simulink model "sldv_property2"  (R2015b)
settings: Solver=FixedStepDiscrete  SolverMode=SingleTasking  StartTime=0.0  StopTime=10.0  RelTol=1e-3
libraries: sldvlib x1
Description:
  | Model Coverage Test Generation
settings Model: Creator=The MathWorks Inc.  LastModifiedBy=amatsumo
settings DataIOCC: SaveFormat=Array  SignalLoggingSaveFormat=ModelDataLogs  SaveOutput=off  SignalLogging=off  SaveTime=off
settings OptimizationCC: BlockReduction=off  ConditionallyExecuteInputs=off  DefaultParameterBehavior=Inlined  ExpressionDepthLimit=2147483647  InitFltsAndDblsToZero=on  EfficientMapNaN2IntZero=off
settings DebuggingCC: AlgebraicLoopMsg=error  SaveWithParameterizedLinksMsg=none  UnderspecifiedInitializationDetection=Classic  MergeDetectMultiDrivingBlocksExec=none  SignalResolutionControl=TryResolveAllWithWarning  SolverPrmCheckMsg=warning  SingleTaskRateTransMsg=error  FcnCallInpInsideContextMsg=UseLocalSettings  StateNameClashWarn=warning
settings HardwareCC: ProdBitPerPointer=32  ProdLargestAtomicFloat=None  ProdIntDivRoundTo=Undefined  ProdEndianess=Unspecified  ProdWordSize=32  ProdHWDeviceType=ASIC/FPGA->ASIC/FPGA  ProdEqTarget=off
settings SFSimCC: SimParseCustomCode=off
settings GRTTargetCC: TargetFcnLib=ansi_tfl_tmw.mat  GeneratePreprocessorConditionals=Disable all  CombineOutputUpdateFcns=off  GRTInterface=on
settings ConfigComp: RecordCoverage=on  CovModelRefEnable=Off  CovSFcnEnable=off  DVMaxProcessTime=60  DVDisplayUnsatisfiableObjectives=on  DVAutomaticStubbing=off  DVMakeOutputFilesUnique=off  DVParameters=on  DVModelCoverageObjectives=MCDC  DVMaxTestCaseSteps=500  DVTestSuiteOptimization=CombinedObjectives  DVAssertions=EnableAll  DVProofAssumptions=EnableAll  DVDetectActiveLogic=on  DVSaveHarnessModel=on  DVModelReferenceHarness=on  DVSaveReport=on  DVActiveTab=4

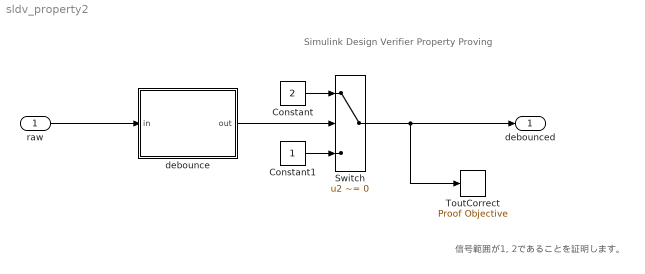
== system sldv_property2 ==
  note: Simulink Design Verifier
      | Property Proving
  note: 信号範囲が1, 2であることを証明します。
  raw : Inport  OutDataTypeStr=boolean
  Constant : Constant  Value=2  OutDataTypeStr=uint8
  Constant1 : Constant  OutDataTypeStr=uint8
  Switch : Switch  Criteria=u2 ~= 0
  ToutCorrect : sldvlib/Objectives and Constraints/Proof Objective  enabled=on  customAVTBlockType=Proof Objective  intervals={1, 2}  dispValues=on  outEnabled=off  enableStopSim=off
      settings: AttributesFormatString=%<intervals>
  debounce : Stateflow chart  TreatAsAtomicUnit=on
  debounced : Outport  OutDataTypeStr=uint8
  wires:
  raw/1 -> debounce/1(in)
  debounce/1(out) -> Switch/2
  Switch/1 -> debounced/1, ToutCorrect/1
  Constant/1 -> Switch/1
  Constant1/1 -> Switch/3

== stateflow chart sldv_property2/debounce ==
  settings: updateMethod=DISCRETE  sampleTime=0.01  stateMachineType=MOORE_MACHINE  executeAtInitialization=1  initializeOutput=1
  state Off
    out = 0;
  state On
    out = 1;
  (default) -> Off
  Off -> On : [in==1]
  On -> Off : [in==0]
  data: in input boolean; out output boolean
